simulink model "rigid_rod_pendulum"  (R2016a)
settings: Solver=ode23  StartTime=0.0  StopTime=10  RelTol=1e-4
undefined symbols (not defined in the file or in its folder): K, magnitude
settings Model: Creator=Aniket  LastModifiedBy=Aniket

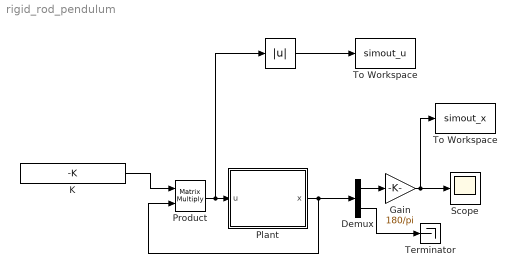
== system rigid_rod_pendulum ==
  "   " : Abs
  Demux : Demux  Outputs=2
  Gain : Gain  Gain=180/pi
  K : Constant  Value=-K  VectorParams1D=off
  Plant : Subsystem
  Product : Product  Multiplication=Matrix(*)
  Scope : Scope
  Terminator : Terminator
  To Workspace : ToWorkspace  VariableName=simout_u  SaveFormat=Structure With Time  SampleTime=-1
  "To Workspace " : ToWorkspace  VariableName=simout_x  SaveFormat=Structure With Time  SampleTime=-1
  wires:
  Demux/1 -> Gain/1
  Gain/1 -> "To Workspace "/1, Scope/1
  Plant/1(x) -> Product/2, Demux/1
  K/1 -> Product/1
  Product/1 -> "   "/1, Plant/1(u)
  Demux/2 -> Terminator/1
  "   "/1 -> To Workspace/1

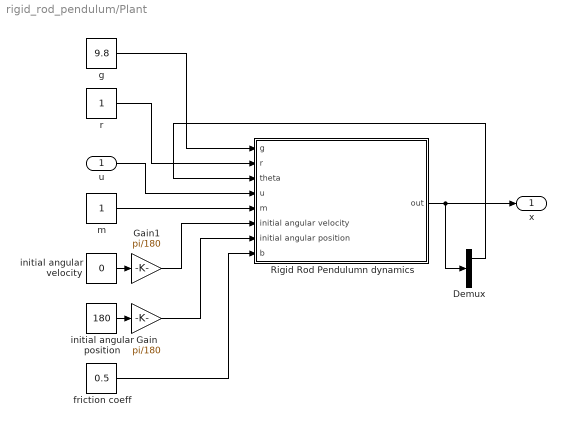
== system rigid_rod_pendulum/Plant ==
  u : Inport  PortDimensions=[1,1]
  Demux : Demux  Outputs=2
  Gain : Gain  Gain=pi/180
  Gain1 : Gain  Gain=pi/180
  Rigid Rod Pendulumn dynamics : Subsystem
  friction coeff : Constant  Value=0.5
  g : Constant  Value=9.8
  initial angular position : Constant  Value=180
  initial angular velocity : Constant  Value=0
  m : Constant
  r : Constant
  x : Outport  PortDimensions=[2 1]
  wires:
  g/1 -> Rigid Rod Pendulumn dynamics/1(g)
  r/1 -> Rigid Rod Pendulumn dynamics/2(r)
  m/1 -> Rigid Rod Pendulumn dynamics/5(m)
  initial angular position/1 -> Gain/1
  u/1 -> Rigid Rod Pendulumn dynamics/4(u)
  friction coeff/1 -> Rigid Rod Pendulumn dynamics/8(b)
  Rigid Rod Pendulumn dynamics/1(out) -> Demux/1, x/1
  Demux/1 -> Rigid Rod Pendulumn dynamics/3(theta)
  Gain/1 -> Rigid Rod Pendulumn dynamics/7(initial angular position)
  initial angular velocity/1 -> Gain1/1
  Gain1/1 -> Rigid Rod Pendulumn dynamics/6(initial angular velocity)

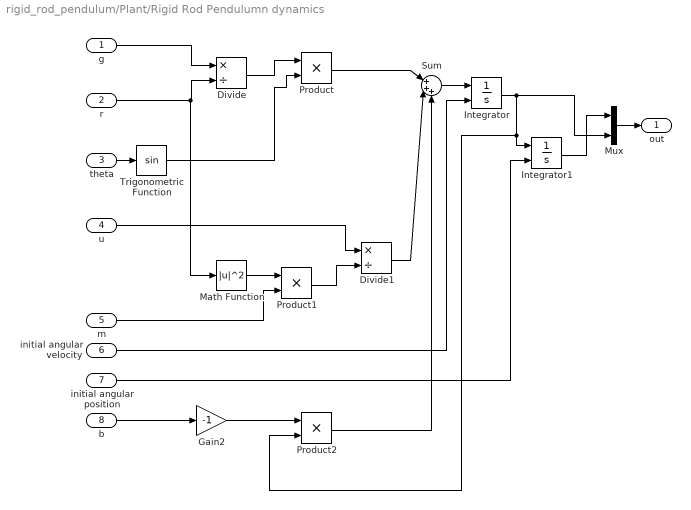
== system rigid_rod_pendulum/Plant/Rigid Rod Pendulumn dynamics ==
  g : Inport
  r : Inport  Port=2
  theta : Inport  Port=3
  u : Inport  Port=4
  m : Inport  Port=5
  initial angular velocity : Inport  Port=6
  initial angular position : Inport  Port=7
  b : Inport  Port=8
  Divide : Product  Inputs=*/
  Divide1 : Product  Inputs=*/
  Gain2 : Gain  Gain=-1
  Integrator : Integrator  InitialConditionSource=external
  Integrator1 : Integrator  InitialConditionSource=external
  Math Function : Math  Operator=magnitude^2  SaturateOnIntegerOverflow=on
  Mux : Mux  Inputs=2
  Product : Product
  Product1 : Product
  Product2 : Product
  Sum : Sum  Inputs=|+++
  Trigonometric Function : Trigonometry
  out : Outport
  wires:
  Product/1 -> Sum/1
  Sum/1 -> Integrator/1
  theta/1 -> Trigonometric Function/1
  Math Function/1 -> Product1/1
  m/1 -> Product1/2
  Trigonometric Function/1 -> Product/2
  u/1 -> Divide1/1
  Divide/1 -> Product/1
  g/1 -> Divide/1
  r/1 -> Math Function/1, Divide/2
  Product1/1 -> Divide1/2
  Integrator/1 -> Product2/2, Integrator1/1, Mux/2
  Divide1/1 -> Sum/2
  initial angular velocity/1 -> Integrator/2
  initial angular position/1 -> Integrator1/2
  b/1 -> Gain2/1
  Gain2/1 -> Product2/1
  Product2/1 -> Sum/3
  Integrator1/1 -> Mux/1
  Mux/1 -> out/1
